simulink model "realmodel_lqr_2016b"  (R2016b)
settings: Solver=ode45  StartTime=0.0  StopTime=10  RelTol=1e-3  EnableMultiTasking=on
values from neighbouring files (symbols this model uses):
  A_eq1_d = sysd1.A    [lin_discr_model.m]    (also in lin_discr_model_test.m)
  B_eq1_d = sysd1.B    [lin_discr_model.m]    (also in lin_discr_model_test.m)
  C_eq1_d = sysd1.C    [lin_discr_model.m]    (also in lin_discr_model_test.m)
  L = place(A_eq1_d',C_eq1_d',pdes)'    [lin_discr_model.m]
  Ts = 0.01    [lin_discr_model.m]    (also in lin_discr_model_test.m)
undefined symbols (not defined in the file or in its folder): adingain, adinoffs, daoutgain, daoutoffs, K12
undefined symbols (not defined in the file): h
settings Model: Creator=rbabuska  LastModifiedBy=jessi
settings DataIOCC: LimitDataPoints=on  SaveFormat=Array  SignalLoggingName=sigsOut
settings OptimizationCC: BooleanDataType=off  ExpressionDepthLimit=2147483647  InitFltsAndDblsToZero=on  LifeSpan=inf
settings DebuggingCC: SaveWithParameterizedLinksMsg=none  SignalResolutionControl=TryResolveAllWithWarning  MultiTaskDSMMsg=warning  MultiTaskCondExecSysMsg=none  AllowSymbolicDim=off  StateNameClashWarn=warning  SFUnexpectedBacktrackingDiag=warning  SFNoUnconditionalDefaultTransitionDiag=warning  SFExecutionAtInitializationDiag=none
settings HardwareCC: ProdBitPerPointer=32  ProdBitPerSizeT=32  ProdBitPerPtrDiffT=32  ProdLargestAtomicFloat=None  ProdIntDivRoundTo=Undefined  ProdEndianess=Unspecified  ProdWordSize=32  ProdHWDeviceType=32-bit Generic  TargetUnknown=on
settings ModelReferenceCC: PropagateSignalLabelsOutOfModel=off
settings GRTTargetCC: TargetFcnLib=ansi_tfl_tmw.mat  TargetLangStandard=C89/C90 (ANSI)  GeneratePreprocessorConditionals=Disable all  CombineOutputUpdateFcns=off  GRTInterface=on
settings ConfigComp: CovMetricSettings=dw  CovHtmlReporting=on  CovSaveCumulativeToWorkspaceVar=on  CovSaveSingleToWorkspaceVar=on  CovExternalEMLEnable=off

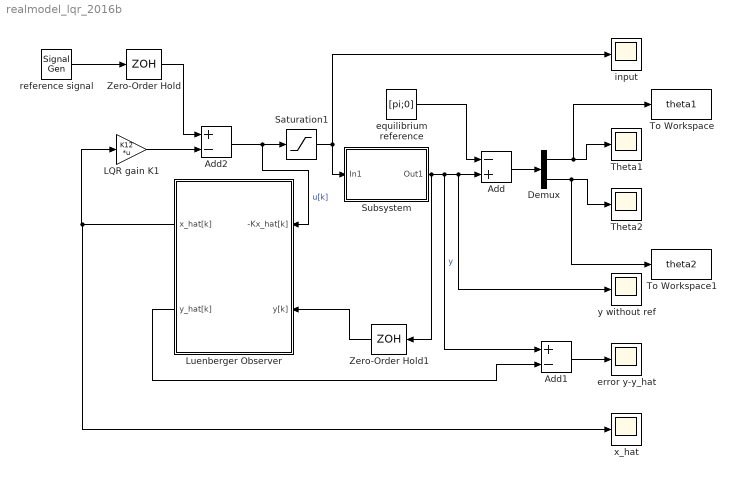
== system realmodel_lqr_2016b ==
  Add : Sum  Inputs=-+
  Add1 : Sum  Inputs=+-
  Add2 : Sum  Inputs=+-
  Demux : Demux  Outputs=2
  LQR gain K1 : Gain  Gain=K12  Multiplication=Matrix(K*u)
  Luenberger Observer : Subsystem
  Saturation1 : Saturate  UpperLimit=1  LowerLimit=-1
  Subsystem : Subsystem
      mask Display: disp('Rotational\nPendulum')
  Theta1 : Scope
  Theta2 : Scope
  To Workspace : ToWorkspace  VariableName=theta1  SaveFormat=Timeseries  SampleTime=-1
  To Workspace1 : ToWorkspace  VariableName=theta2  SaveFormat=Timeseries  SampleTime=-1
  Zero-Order Hold : ZeroOrderHold  SampleTime=Ts
  Zero-Order Hold1 : ZeroOrderHold  SampleTime=Ts
  equilibrium reference : Constant  Value=[pi;0]
  error y-y_hat : Scope
  input : Scope
  reference signal : SignalGenerator  WaveForm=square  Amplitude=-0.3
  x_hat : Scope
  y without ref : Scope
  wires:
  Saturation1/1 -> Subsystem/1(In1), input/1
  Demux/1 -> To Workspace/1, Theta1/1
  Demux/2 -> To Workspace1/1, Theta2/1
  Subsystem/1(Out1) -> Add1/1, y without ref/1, Add/2, Zero-Order Hold1/1  "y"
  Add/1 -> Demux/1
  equilibrium reference/1 -> Add/1
  Add2/1 -> Luenberger Observer/1(-Kx_hat[k]), Saturation1/1  "u[k]"
  LQR gain K1/1 -> Add2/2
  reference signal/1 -> Zero-Order Hold/1
  Zero-Order Hold/1 -> Add2/1
  Luenberger Observer/1(x_hat[k]) -> x_hat/1, LQR gain K1/1
  Zero-Order Hold1/1 -> Luenberger Observer/2(y[k])
  Luenberger Observer/2(y_hat[k]) -> Add1/2
  Add1/1 -> error y-y_hat/1

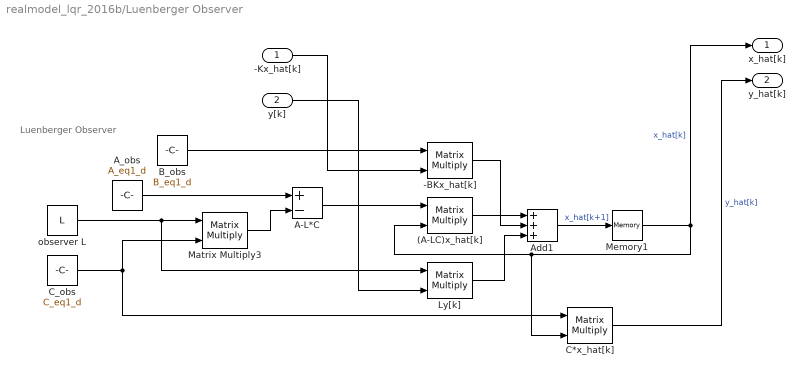
== system realmodel_lqr_2016b/Luenberger Observer ==
  note: Luenberger Observer
  -Kx_hat[k] : Inport
  y[k] : Inport  Port=2
  (A-LC)x_hat[k] : Product  Multiplication=Matrix(*)
  -BKx_hat[k] : Product  Multiplication=Matrix(*)
  A-L*C : Sum  Inputs=+-
  A_obs : Constant  Value=A_eq1_d  SampleTime=Ts
  Add1 : Sum  Inputs=+++
  B_obs : Constant  Value=B_eq1_d  SampleTime=Ts
  C*x_hat[k] : Product  Multiplication=Matrix(*)
  C_obs : Constant  Value=C_eq1_d  SampleTime=Ts
  Ly[k] : Product  Multiplication=Matrix(*)
  Matrix Multiply3 : Product  Multiplication=Matrix(*)
  Memory1 : Memory  X0=[pi; 0;0;0]
  observer L : Constant  Value=L  SampleTime=Ts
  x_hat[k] : Outport
  y_hat[k] : Outport  Port=2
  wires:
  (A-LC)x_hat[k]/1 -> Add1/1
  A-L*C/1 -> (A-LC)x_hat[k]/1
  Add1/1 -> Memory1/1  "x_hat[k+1]"
  observer L/1 -> Ly[k]/1, Matrix Multiply3/1
  C_obs/1 -> C*x_hat[k]/1, Matrix Multiply3/2
  Ly[k]/1 -> Add1/3
  Matrix Multiply3/1 -> A-L*C/2
  A_obs/1 -> A-L*C/1
  Memory1/1 -> C*x_hat[k]/2, (A-LC)x_hat[k]/2, x_hat[k]/1  "x_hat[k]"
  y[k]/1 -> Ly[k]/2
  C*x_hat[k]/1 -> y_hat[k]/1  "y_hat[k]"
  -Kx_hat[k]/1 -> -BKx_hat[k]/2
  B_obs/1 -> -BKx_hat[k]/1
  -BKx_hat[k]/1 -> Add1/2

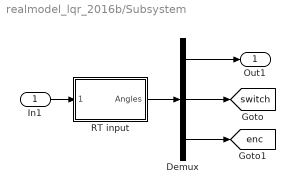
== system realmodel_lqr_2016b/Subsystem ==
  In1 : Inport
  Demux : Demux  Outputs=[2 4 1]
  RT input : Subsystem  mask{Ts=h, channels=[6 7]}
      mask prompts: Ts "Sample time [s]:"; channels "Channels to read (e.g., [6 7])"
      mask init:
      | hwinit;
      | 
      | % initialize FPGA
      | fugihandle = fugiboard('Open', 'Pendulum1');
      | fugihandle.WatchdogTimeout = 0.5;
      | fugiboard('SetParams', fugihandle);
      | fugiboard('Write', fugihandle, 0, 0, 0, 0);  % dummy write to sync interface board
      | fugiboard('Write', fugihandle, 5, 1, 0, 0);  % reset position, activate relay
      | data = fugiboard('Read', fugihandle);        % get version info from FPGA
      | % model = bitshift(data(1), -5); 
      | % version = bitand(data(1), 31);
      | % disp(sprintf('FPGA setup %d, version %d', model, version)); % for the B&P it should say 1 1, or else there is a problem
      | fugiboard('Write', fugihandle, 0, 1, 0, 0);  % end reset
      | pause(0.1);                         % give relay some time to respond
      mask Display: disp('Rotational\nPendulum')
  Out1 : Outport
  tag scope: enc=global, switch=global
  wires:
  RT input/1(Angles) -> Demux/1
  Demux/1 -> Out1/1
  Demux/2 -> [switch]
  Demux/3 -> [enc]
  In1/1 -> RT input/1(Motors)

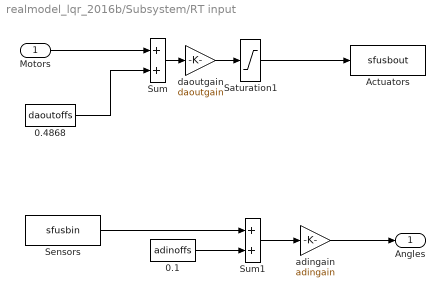
== system realmodel_lqr_2016b/Subsystem/RT input ==
  Motors : Inport
  0.1 : Constant  Value=adinoffs
  0.4868 : Constant  Value=daoutoffs
  Actuators : S-Function  FunctionName=sfusbout  Parameters=Ts, fugihandle  SFunctionDeploymentMode=off  EnableBusSupport=off
  Saturation1 : Saturate  UpperLimit=10  LowerLimit=-10
  Sensors : S-Function  FunctionName=sfusbin  Parameters=Ts, fugihandle, channels  SFunctionDeploymentMode=off  EnableBusSupport=off
  Sum : Sum  SaturateOnIntegerOverflow=on  InputSameDT=on  OutDataTypeStr=Inherit: Same as first input
  Sum1 : Sum  SaturateOnIntegerOverflow=on  InputSameDT=on  OutDataTypeStr=Inherit: Same as first input
  adingain : Gain  Gain=adingain  SaturateOnIntegerOverflow=on  OutDataTypeStr=Inherit: Same as input  ParamDataTypeStr=Inherit: Same as input
  daoutgain : Gain  Gain=daoutgain  SaturateOnIntegerOverflow=on  OutDataTypeStr=Inherit: Same as input  ParamDataTypeStr=Inherit: Same as input
  Angles : Outport
  wires:
  Sum/1 -> daoutgain/1
  0.4868/1 -> Sum/2
  Motors/1 -> Sum/1
  Sum1/1 -> adingain/1
  0.1/1 -> Sum1/2
  adingain/1 -> Angles/1
  Saturation1/1 -> Actuators/1
  daoutgain/1 -> Saturation1/1
  Sensors/1 -> Sum1/1
